simulink model "Trafficlight"  (R2023a)
settings: Solver=VariableStepAuto  StartTime=0.0  StopTime=10.0  RelTol=1e-3
settings Model: Creator=Egypt_Laptop  LastModifiedBy=Egypt_Laptop

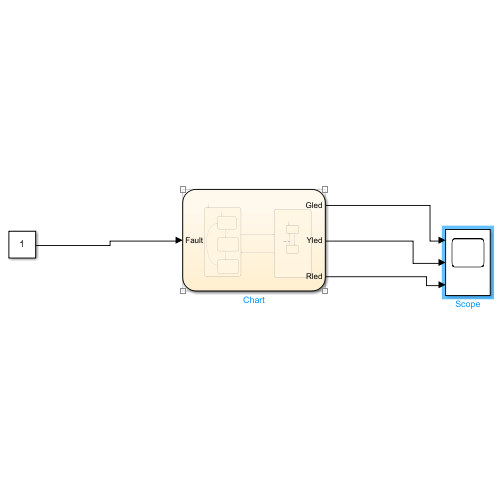
[thumbnail: Simulink's stored preview of the top-level diagram]
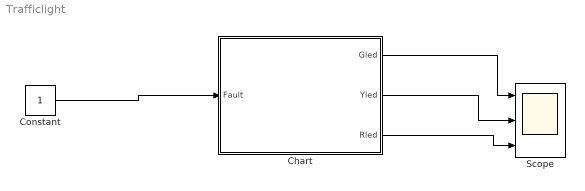
== system Trafficlight ==
  Chart : Stateflow chart  TreatAsAtomicUnit=on
  Constant : Constant
  Scope : Scope  NumInputPorts=3
  wires:
  Chart/1(Gled) -> Scope/1
  Chart/2(Yled) -> Scope/2
  Chart/3(Rled) -> Scope/3
  Constant/1 -> Chart/1(Fault)

== stateflow chart Trafficlight/Chart ==
  state NormalMode
    state stop
      en:
      Rled =1;
      %Yled=0;
      %Gled=0;
      ex:
      Rled=0;
    state GO
      en:
      %Rled =0;
      %Yled=0;
      Gled=1;
      ex:
      Gled=0;
    state PTS
      en:
      %Rled =0;
      Yled=1;
      %Gled=0;
      ex:
      Yled=0;
    (default) -> stop
    PTS -> stop : after(1,sec)
    stop -> GO : after(1,sec)
    GO -> PTS : after(1,sec)
  state FaultMode
    state ON
      en:
      Rled=1;
    note: after ( 1 , sec )
    state OFF
      en:
      Rled=0;
    (default) -> ON
    OFF -> ON
    ON -> OFF : after(1,sec)
  (default) -> NormalMode
  NormalMode -> FaultMode : [Fault==1]
  FaultMode -> NormalMode : [Fault==0]
  data: Gled output; Yled output; Rled output; Fault input
